simulink model "vhs_fpga_rx_to_sdram_time_share_agc_cfo"  (Simulink 7.1)
settings: Solver=FixedStepDiscrete  SolverMode=SingleTasking  StartTime=0.0  StopTime=inf  RelTol=1e-3
values from neighbouring files (symbols this model uses):
  N_FB_RX_frame = 390    [OFDM_Parameter.mat]
  Nfft = 64    [OFDM_Parameter.mat]
  Nguard = 16    [OFDM_Parameter.mat]
  Nofdm = 130    [OFDM_Parameter.mat]
  Nskip = 8    [OFDM_Parameter.mat]
undefined symbols (not defined in the file or in its folder): Fs, Sincos_Bits, Sincos_Len, Theta_Bits
libraries: xbsIndex_r4 x366, vhsadac_common_ob_fpgalib_v1_2_0 x18, misc_tools_fpgalib_v1_0_0 x6, rffe_fpgalib_v1_1_0 x1, rtdex_fpgalib_v1_1_0 x1
(part 1 of 5)
settings Model: Creator=Administrator  LastModifiedBy=lyrtech

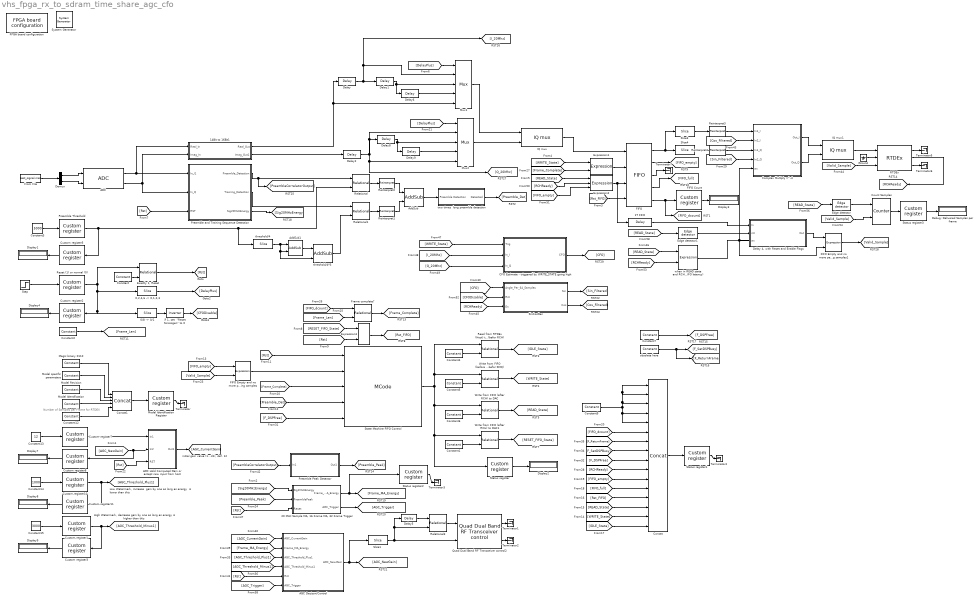
== system vhs_fpga_rx_to_sdram_time_share_agc_cfo ==
  note: Number of Samples per Frame for RTDEX
  " System Generator" : xbsIndex_r4/ System Generator  Tag=genX  SystemSampleTime=-1  xilinxfamily=virtex4  part=xc4vsx55  speed=-10  package=ff1148  synthesis_tool=XST  clock_wrapper=Clock Enables  directory=./netlist  testbench=off  simulink_period=1  sysclk_period=9  dcm_input_clock_period=100  incr_netlist=off  trim_vbits=Everywhere in SubSystem  dbl_ovrd=According to Block Masks  core_generation=According to Block Masks  run_coregen=off  deprecated_control=off  eval_field=0  block_type=sysgen
      settings: block_version=10.1.3
  "0,2,4,6 -> 0,1,2,3" : xbsIndex_r4/Slice  nbits=2  boolean_output=off  mode=Lower Bit Location + Width  bit1=0  base1=MSB of Input  bit0=1  base0=LSB of Input  dbl_ovrd=off  block_type=slice
      settings: infoedit="Extracts a given range of bits from each input sample and presents it at the output.  The output type is ordinarily unsigned with binary point at zero, but can be Boolean when the slice is one bit wide.<P><P>Hardware notes: In hardware this block costs nothing."  block_version=10.1.3
  "0/8 -> 0/1" : xbsIndex_r4/Slice  nbits=1  boolean_output=on  mode=Lower Bit Location + Width  bit1=0  base1=MSB of Input  bit0=3  base0=LSB of Input  dbl_ovrd=off  block_type=slice
      settings: infoedit="Extracts a given range of bits from each input sample and presents it at the output.  The output type is ordinarily unsigned with binary point at zero, but can be Boolean when the slice is one bit wide.<P><P>Hardware notes: In hardware this block costs nothing."  block_version=10.1.3
  14Bit to 16Bit1 : Subsystem
  1T FIFO : xbsIndex_r4/Delay  en=off  latency=1  dbl_ovrd=off  reg_retiming=off  block_type=delay
  "20 MHz Sample MA, 16 Frame MA, 32 Frame Trigger" : Subsystem
  ADC : vhsadac_common_ob_fpgalib_v1_2_0/ADC  Tag=LYR_FPGA_IO_ADC  Description=Lyrtech block  SystemSampleTime=-1  nbofcha=2  binpt=0  sample_period=5  ovr_flag=off  trig_sig=off
  AGC Decison/Control : Subsystem
  AGC Hold Computed Gain or accept new input from host : Subsystem
  AddSub : xbsIndex_r4/AddSub  mode=Addition  use_carryin=off  use_carryout=off  en=off  latency=0  precision=Full  arith_type=Unsigned  n_bits=16  bin_pt=14  quantization=Truncate  overflow=Wrap  dbl_ovrd=off  use_behavioral_HDL=off  pipelined=off  use_rpm=on  hw_selection=Fabric  block_type=addsub
      settings: block_version=10.1.3
  AddSub1 : xbsIndex_r4/AddSub  mode=Addition  use_carryin=off  use_carryout=off  en=off  latency=1  precision=Full  arith_type=Unsigned  n_bits=16  bin_pt=14  quantization=Truncate  overflow=Wrap  dbl_ovrd=off  use_behavioral_HDL=off  pipelined=off  use_rpm=on  hw_selection=Fabric  block_type=addsub
      settings: block_version=10.1.3
  CFO Estimate - triggered by WRITE_STATE going high : Subsystem
  Complex Multiply z^-4 : Subsystem
  Concat : xbsIndex_r4/Concat  num_inputs=16  dbl_ovrd=off  block_type=concat
      settings: block_version=10.1.3
  Concat1 : xbsIndex_r4/Concat  num_inputs=5  dbl_ovrd=off  block_type=concat
      settings: block_version=10.1.3
  Constant : xbsIndex_r4/Constant  arith_type=Unsigned  const=1  n_bits=32  bin_pt=0  explicit_period=on  period=5  equ=P=C  opselect=C  inp2=PCIN>>17  opr=+  inp1=P  carry=CIN  dbl_ovrd=off  block_type=constant
  Constant1 : xbsIndex_r4/Constant  arith_type=Unsigned  const=4  n_bits=3  bin_pt=0  explicit_period=on  period=5  equ=P=C  opselect=C  inp2=PCIN>>17  opr=+  inp1=P  carry=CIN  dbl_ovrd=off  block_type=constant
  Constant12 : xbsIndex_r4/Constant  arith_type=Unsigned  const=N_FB_RX_frame  n_bits=15  bin_pt=0  explicit_period=on  period=1  equ=P=C  opselect=C  inp2=PCIN>>17  opr=+  inp1=P  carry=CIN  dbl_ovrd=off  block_type=constant
  Constant13 : Constant  Value=12  OutDataType=sfix(16)  OutScaling=2^0  SampleTime=5
  Constant14 : Constant  Value=1000  OutDataType=sfix(16)  OutScaling=2^0  SampleTime=5
  Constant15 : Constant  Value=3000  OutDataType=sfix(16)  OutScaling=2^0  SampleTime=5
  Constant2 : xbsIndex_r4/Constant  arith_type=Unsigned  const=(Nfft + Nguard) * ( 1 + Nofdm )  n_bits=32  bin_pt=0  explicit_period=on  period=5  equ=P=C  opselect=C  inp2=PCIN>>17  opr=+  inp1=P  carry=CIN  dbl_ovrd=off  block_type=constant
  Constant3 : Constant  Value=5000  OutDataType=sfix(16)  OutScaling=2^0  SampleTime=5
  Constant4 : xbsIndex_r4/Constant  arith_type=Unsigned  const=1  n_bits=3  bin_pt=0  explicit_period=on  period=5  equ=P=C  opselect=C  inp2=PCIN>>17  opr=+  inp1=P  carry=CIN  dbl_ovrd=off  block_type=constant
  Constant5 : xbsIndex_r4/Constant  arith_type=Unsigned  const=2  n_bits=3  bin_pt=0  explicit_period=on  period=5  equ=P=C  opselect=C  inp2=PCIN>>17  opr=+  inp1=P  carry=CIN  dbl_ovrd=off  block_type=constant
  Constant6 : xbsIndex_r4/Constant  arith_type=Unsigned  const=3  n_bits=3  bin_pt=0  explicit_period=on  period=5  equ=P=C  opselect=C  inp2=PCIN>>17  opr=+  inp1=P  carry=CIN  dbl_ovrd=off  block_type=constant
  Constant7 : xbsIndex_r4/Constant  arith_type=Boolean  const=1  n_bits=3  bin_pt=0  explicit_period=on  period=5  equ=P=C  opselect=C  inp2=PCIN>>17  opr=+  inp1=P  carry=CIN  dbl_ovrd=off  block_type=constant
  Constant9 : xbsIndex_r4/Constant  arith_type=Unsigned  const=0  n_bits=1  bin_pt=0  explicit_period=on  period=5  equ=P=C  opselect=C  inp2=PCIN>>17  opr=+  inp1=P  carry=CIN  dbl_ovrd=off  block_type=constant
  Count Samples : xbsIndex_r4/Counter  cnt_type=Free Running  cnt_to=Inf  operation=Up  start_count=0  cnt_by_val=1  arith_type=Unsigned  n_bits=16  bin_pt=0  load_pin=off  rst=on  en=on  explicit_period=on  period=5  dbl_ovrd=off  use_behavioral_HDL=off  use_rpm=off  implementation=Fabric  block_type=counter
      settings: block_version=VER_STRING_GOES_HERE
  Custom register1 : vhsadac_common_ob_fpgalib_v1_2_0/Custom register  Tag=LYR_FPGA_IO_CUSTOM_REGISTER  Description=Lyrtech block  SystemSampleTime=-1  regID=10  direction=Read  output_arithmetic_type=Unsigned  output_width=32  binpt=0  sample_period=5
  Custom register10 : vhsadac_common_ob_fpgalib_v1_2_0/Custom register  Tag=LYR_FPGA_IO_CUSTOM_REGISTER  Description=Lyrtech block  SystemSampleTime=-1  regID=9  direction=Read  output_arithmetic_type=Unsigned  output_width=32  binpt=0  sample_period=5
  Custom register11 : vhsadac_common_ob_fpgalib_v1_2_0/Custom register  Tag=LYR_FPGA_IO_CUSTOM_REGISTER  Description=Lyrtech block  Orientation=left  SystemSampleTime=-1  regID=9  direction=Write  output_arithmetic_type=Unsigned  output_width=32  binpt=0  sample_period=5
  Custom register2 : vhsadac_common_ob_fpgalib_v1_2_0/Custom register  Tag=LYR_FPGA_IO_CUSTOM_REGISTER  Description=Lyrtech block  Orientation=left  SystemSampleTime=-1  regID=2  direction=Write  output_arithmetic_type=Unsigned  output_width=32  binpt=0  sample_period=5
  Custom register3 : vhsadac_common_ob_fpgalib_v1_2_0/Custom register  Tag=LYR_FPGA_IO_CUSTOM_REGISTER  Description=Lyrtech block  Orientation=left  SystemSampleTime=-1  regID=10  direction=Write  output_arithmetic_type=Unsigned  output_width=32  binpt=0  sample_period=5
  Custom register5 : vhsadac_common_ob_fpgalib_v1_2_0/Custom register  Tag=LYR_FPGA_IO_CUSTOM_REGISTER  Description=Lyrtech block  Orientation=left  SystemSampleTime=-1  regID=1  direction=Write  output_arithmetic_type=Unsigned  output_width=32  binpt=0  sample_period=5
  Custom register7 : vhsadac_common_ob_fpgalib_v1_2_0/Custom register  Tag=LYR_FPGA_IO_CUSTOM_REGISTER  Description=Lyrtech block  SystemSampleTime=-1  regID=8  direction=Read  output_arithmetic_type=Unsigned  output_width=32  binpt=0  sample_period=5
  Custom register8 : vhsadac_common_ob_fpgalib_v1_2_0/Custom register  Tag=LYR_FPGA_IO_CUSTOM_REGISTER  Description=Lyrtech block  Orientation=left  SystemSampleTime=-1  regID=8  direction=Write  output_arithmetic_type=Unsigned  output_width=32  binpt=0  sample_period=5
  Debug: Delivered Samples per frame : Display
  Delay : xbsIndex_r4/Delay  en=off  latency=106  dbl_ovrd=off  reg_retiming=off  block_type=delay
  "Delay 4, with Reset and Enable Flags" : Subsystem
  Delay{1,5..6,8..9} (5 alike) : xbsIndex_r4/Delay  en=off  latency=1  dbl_ovrd=off  reg_retiming=off  block_type=delay
  Delay2 : xbsIndex_r4/Delay  en=off  latency=106  dbl_ovrd=off  reg_retiming=off  block_type=delay
  Demux : Demux  Outputs=2
  Display{1..4,7..9} (7 alike) : Display
  Edge detector : misc_tools_fpgalib_v1_0_0/Edge detector  Tag=LYR_FPGA_MISC_EDGE_DETECTOR  Description=Lyrtech block  SystemSampleTime=-1  edge_detect=Rising  and_latency=0
  Edge detector1 : misc_tools_fpgalib_v1_0_0/Edge detector  Tag=LYR_FPGA_MISC_EDGE_DETECTOR  Description=Lyrtech block  SystemSampleTime=-1  edge_detect=Rising  and_latency=0
  "Exactly 1, Reset" : xbsIndex_r4/Relational  mode=a=b  en=off  latency=1  dbl_ovrd=off  block_type=relational
      settings: block_version=10.1.3
  Expression1 : xbsIndex_r4/Expression  expression=a & ~b  align_bp=on  en=off  latency=0  precision=Full  arith_type=Unsigned  n_bits=16  bin_pt=0  dbl_ovrd=off  block_type=expr
      settings: block_version=10.1.3
  Expression2 : xbsIndex_r4/Expression  expression=a & b & ~c  align_bp=on  en=off  latency=0  precision=Full  arith_type=Unsigned  n_bits=16  bin_pt=0  dbl_ovrd=off  block_type=expr
      settings: block_version=10.1.3
  Expression3 : xbsIndex_r4/Expression  expression=a | b  align_bp=on  en=off  latency=0  precision=Full  arith_type=Unsigned  n_bits=16  bin_pt=0  dbl_ovrd=off  block_type=expr
      settings: block_version=10.1.3
  FIFO : xbsIndex_r4/FIFO  depth=16K  percent_nbits=1  rst=on  en=off  use_dcount=on  use_almost_empty=off  almost_empty_thresh=2  use_almost_full=off  almost_full_thresh=14  dbl_ovrd=off  mem_type=Block RAM  block_type=fifo
      settings: block_version=10.1.3
  FIFO Count : vhsadac_common_ob_fpgalib_v1_2_0/Custom register  Tag=LYR_FPGA_IO_CUSTOM_REGISTER  Description=Lyrtech block  SystemSampleTime=-1  regID=3  direction=Write  output_arithmetic_type=Unsigned  output_width=32  binpt=0  sample_period=5
  FIFO Empty and no more pending samples : xbsIndex_r4/Expression  expression=a & ~b  align_bp=on  en=off  latency=0  precision=Full  arith_type=Unsigned  n_bits=16  bin_pt=0  dbl_ovrd=off  block_type=expr
      settings: block_version=10.1.3
  FIFO Empty and no more pending samples1 : xbsIndex_r4/Expression  expression=a & b  align_bp=on  en=off  latency=0  precision=Full  arith_type=Unsigned  n_bits=16  bin_pt=0  dbl_ovrd=off  block_type=expr
      settings: block_version=10.1.3
  FPGA board configuration : vhsadac_common_ob_fpgalib_v1_2_0/FPGA board configuration  Tag=SysgenCompile  Description=Lyrtech block  SystemSampleTime=-1  clk_sel=Hardware implementation  clk_src=ADC/DAC clock  hardware=VHS-ADC Virtex-4  copy_bit_cd=on
  Frame complete? : xbsIndex_r4/Relational  mode=a>=b  en=off  latency=0  dbl_ovrd=off  block_type=relational
      settings: block_version=10.1.3
  From File : FromFile  FileName=test_signal.mat  SampleTime=5
  Ground : Ground
  IQ mux : misc_tools_fpgalib_v1_0_0/IQ mux  Tag=LYR_FPGA_MISC_IQ_MUX  Description=Lyrtech block  SystemSampleTime=-1
  IQ mux1 : misc_tools_fpgalib_v1_0_0/IQ mux  Tag=LYR_FPGA_MISC_IQ_MUX  Description=Lyrtech block  SystemSampleTime=-1
  Magic binary 0110 : xbsIndex_r4/Constant  arith_type=Unsigned  const=6  n_bits=4  bin_pt=0  explicit_period=on  period=1  equ=P=C  opselect=C  inp2=PCIN>>17  opr=+  inp1=P  carry=CIN  dbl_ovrd=off  block_type=constant
  Model Identification : xbsIndex_r4/Constant  arith_type=Unsigned  const=1  n_bits=4  bin_pt=0  explicit_period=on  period=1  equ=P=C  opselect=C  inp2=PCIN>>17  opr=+  inp1=P  carry=CIN  dbl_ovrd=off  block_type=constant
  Model Identification Register : vhsadac_common_ob_fpgalib_v1_2_0/Custom register  Tag=LYR_FPGA_IO_CUSTOM_REGISTER  Description=Lyrtech block  SystemSampleTime=-1  regID=7  direction=Write  output_arithmetic_type=Unsigned  output_width=32  binpt=0  sample_period=1
  Model Revision : xbsIndex_r4/Constant  arith_type=Unsigned  const=2  n_bits=3  bin_pt=0  explicit_period=on  period=1  equ=P=C  opselect=C  inp2=PCIN>>17  opr=+  inp1=P  carry=CIN  dbl_ovrd=off  block_type=constant
  Model specific parameters : xbsIndex_r4/Constant  arith_type=Unsigned  const=0  n_bits=6  bin_pt=0  explicit_period=on  period=1  equ=P=C  opselect=C  inp2=PCIN>>17  opr=+  inp1=P  carry=CIN  dbl_ovrd=off  block_type=constant
  Mux1 : xbsIndex_r4/Mux  inputs=4  en=off  latency=0  precision=Full  arith_type=Unsigned  n_bits=16  bin_pt=14  quantization=Truncate  overflow=Wrap  dbl_ovrd=off  block_type=mux
  Mux2 : xbsIndex_r4/Mux  inputs=4  en=off  latency=0  precision=Full  arith_type=Unsigned  n_bits=16  bin_pt=14  quantization=Truncate  overflow=Wrap  dbl_ovrd=off  block_type=mux
  Preamble Peak Detector : Subsystem
  Preamble Threshold : vhsadac_common_ob_fpgalib_v1_2_0/Custom register  Tag=LYR_FPGA_IO_CUSTOM_REGISTER  Description=Lyrtech block  SystemSampleTime=-1  regID=1  direction=Read  output_arithmetic_type=Unsigned  output_width=32  binpt=0  sample_period=5
  Preamble and Training Sequence Detection : Subsystem
  Quad Dual Band RF Transceiver control2 : rffe_fpgalib_v1_1_0/Quad Dual Band RF Transceiver control  Tag=LYR_FPGA_CONTROL_QUAD_DUAL_BAND_RF_TRANSCEIVER_CONTROL  Description=Lyrtech block  SystemSampleTime=-1  external_gain=on  tx1=off  tx2=off  tx3=off  tx4=off  mode=off  add=off  int_divider=off  frac_divider=off  int_divider_en=off  frac_divider_en=off  lock_detect=off  sample_period=5
  RTDEx : rtdex_fpgalib_v1_1_0/RTDEx  Tag=LYR_FPGA_IO_RTDEX  Description=Lyrtech block  SystemSampleTime=-1  direction=TX  output_arithmetic_type=Unsigned  output_width=32  binpt=0  provide_control=off  sample_period=5
  Read from RTDEx (Host) to FIFO (befor RCH) : xbsIndex_r4/Relational  mode=a=b  en=off  latency=0  dbl_ovrd=off  block_type=relational
      settings: block_version=10.1.3
  Reinterpret1 : xbsIndex_r4/Reinterpret  force_arith_type=on  arith_type=Unsigned  force_bin_pt=on  bin_pt=0  block_type=reinterpret
      settings: infoedit="Changes signal type without altering the binary representation.   You can changed the signal between signed and unsigned, and relocate the binary point.<P><P>Hardware notes: In hardware this block costs nothing.<P><P>Example:  Suppose the input is 6 bits wide, signed, with 2 fractional bits, and the output is forced to unsigned with 0 fractional bits.  Then an input of -2.0 (1110.00 in binary 2's complement) becomes an output of 56 (111000 in binary)."  block_version=10.1.3
  Reinterpret2 : xbsIndex_r4/Reinterpret  force_arith_type=on  arith_type=Unsigned  force_bin_pt=on  bin_pt=0  block_type=reinterpret
      settings: infoedit="Changes signal type without altering the binary representation.   You can changed the signal between signed and unsigned, and relocate the binary point.<P><P>Hardware notes: In hardware this block costs nothing.<P><P>Example:  Suppose the input is 6 bits wide, signed, with 2 fractional bits, and the output is forced to unsigned with 0 fractional bits.  Then an input of -2.0 (1110.00 in binary 2's complement) becomes an output of 56 (111000 in binary)."  block_version=10.1.3
  Reinterpret3 : xbsIndex_r4/Reinterpret  force_arith_type=on  arith_type="Signed  (2's comp)"  force_bin_pt=on  bin_pt=0  block_type=reinterpret
      settings: infoedit="Changes signal type without altering the binary representation.   You can changed the signal between signed and unsigned, and relocate the binary point.<P><P>Hardware notes: In hardware this block costs nothing.<P><P>Example:  Suppose the input is 6 bits wide, signed, with 2 fractional bits, and the output is forced to unsigned with 0 fractional bits.  Then an input of -2.0 (1110.00 in binary 2's complement) becomes an output of 56 (111000 in binary)."  block_version=10.1.3
  Reinterpret4 : xbsIndex_r4/Reinterpret  force_arith_type=on  arith_type="Signed  (2's comp)"  force_bin_pt=on  bin_pt=0  block_type=reinterpret
      settings: infoedit="Changes signal type without altering the binary representation.   You can changed the signal between signed and unsigned, and relocate the binary point.<P><P>Hardware notes: In hardware this block costs nothing.<P><P>Example:  Suppose the input is 6 bits wide, signed, with 2 fractional bits, and the output is forced to unsigned with 0 fractional bits.  Then an input of -2.0 (1110.00 in binary 2's complement) becomes an output of 56 (111000 in binary)."  block_version=10.1.3
  Relational : xbsIndex_r4/Relational  mode=a>=b  en=off  latency=1  dbl_ovrd=off  block_type=relational
      settings: block_version=10.1.3
  Relational1 : xbsIndex_r4/Relational  mode=a>=b  en=off  latency=1  dbl_ovrd=off  block_type=relational
      settings: block_version=10.1.3
  Relational3 : xbsIndex_r4/Relational  mode=a!=b  en=off  latency=1  dbl_ovrd=off  block_type=relational
      settings: block_version=10.1.3
  Reset (1) or normal (0) : vhsadac_common_ob_fpgalib_v1_2_0/Custom register  Tag=LYR_FPGA_IO_CUSTOM_REGISTER  Description=Lyrtech block  SystemSampleTime=-1  regID=2  direction=Read  output_arithmetic_type=Unsigned  output_width=32  binpt=0  sample_period=5
  SinCosGen : Subsystem
  Slice1 : xbsIndex_r4/Slice  nbits=7  boolean_output=off  mode=Lower Bit Location + Width  bit1=0  base1=MSB of Input  bit0=0  base0=LSB of Input  dbl_ovrd=off  block_type=slice
      settings: infoedit="Extracts a given range of bits from each input sample and presents it at the output.  The output type is ordinarily unsigned with binary point at zero, but can be Boolean when the slice is one bit wide.<P><P>Hardware notes: In hardware this block costs nothing."  block_version=10.1.3
  Slice3 : xbsIndex_r4/Slice  nbits=16  boolean_output=off  mode=Upper Bit Location + Width  bit1=0  base1=MSB of Input  bit0=0  base0=LSB of Input  dbl_ovrd=off  block_type=slice
      settings: infoedit="Extracts a given range of bits from each input sample and presents it at the output.  The output type is ordinarily unsigned with binary point at zero, but can be Boolean when the slice is one bit wide.<P><P>Hardware notes: In hardware this block costs nothing."  block_version=10.1.3
  Slice4 : xbsIndex_r4/Slice  nbits=16  boolean_output=off  mode=Lower Bit Location + Width  bit1=0  base1=MSB of Input  bit0=0  base0=LSB of Input  dbl_ovrd=off  block_type=slice
      settings: infoedit="Extracts a given range of bits from each input sample and presents it at the output.  The output type is ordinarily unsigned with binary point at zero, but can be Boolean when the slice is one bit wide.<P><P>Hardware notes: In hardware this block costs nothing."  block_version=10.1.3
  State Machine FIFO Control : xbsIndex_r4/MCode  mfname=vhs_state_machine_fifo  explicit_period=on  period=5  inputsTable={'boundInpExpr'=>['','','','',''],'inputs'=>['RST','FIFO_Empty','FIFO_Filled','Preamble_Det','DSPFree']}  outputsTable={'outputs'=>['sel'],'suppressOut'=>['off']}  dbl_ovrd=off  enable_stdout=off  enable_debug=off  suppress_output=1  defparams={}  hide_port_list={}  block_type=mcode
      settings: block_version=10.1.3
  Status register : vhsadac_common_ob_fpgalib_v1_2_0/Custom register  Tag=LYR_FPGA_IO_CUSTOM_REGISTER  Description=Lyrtech block  SystemSampleTime=-1  regID=0  direction=Write  output_arithmetic_type=Unsigned  output_width=32  binpt=0  sample_period=5
  Status register1 : vhsadac_common_ob_fpgalib_v1_2_0/Custom register  Tag=LYR_FPGA_IO_CUSTOM_REGISTER  Description=Lyrtech block  SystemSampleTime=-1  regID=5  direction=Write  output_arithmetic_type=Unsigned  output_width=32  binpt=0  sample_period=5
  Status register2 : vhsadac_common_ob_fpgalib_v1_2_0/Custom register  Tag=LYR_FPGA_IO_CUSTOM_REGISTER  Description=Lyrtech block  SystemSampleTime=-1  regID=11  direction=Write  output_arithmetic_type=Unsigned  output_width=32  binpt=0  sample_period=5
  Status register3 : vhsadac_common_ob_fpgalib_v1_2_0/Custom register  Tag=LYR_FPGA_IO_CUSTOM_REGISTER  Description=Lyrtech block  SystemSampleTime=-1  regID=6  direction=Write  output_arithmetic_type=Unsigned  output_width=32  binpt=0  sample_period=5
  Step : Step  Time=5  Before=1  After=0  SampleTime=5
  Terminator{,1..7} (8 alike) : Terminator
  Write from FIFO (after RCH) to DAC : xbsIndex_r4/Relational  mode=a=b  en=off  latency=0  dbl_ovrd=off  block_type=relational
      settings: block_version=10.1.3
  Write from FIFO (after RCH) to DAC1 : xbsIndex_r4/Relational  mode=a=b  en=off  latency=0  dbl_ovrd=off  block_type=relational
      settings: block_version=10.1.3
  Write from FIFO (before RCH) to RCH (befor SMQ) : xbsIndex_r4/Relational  mode=a=b  en=off  latency=0  dbl_ovrd=off  block_type=relational
      settings: block_version=10.1.3
  "if 1, set  \"Reset Sincosgen\" to 0" : xbsIndex_r4/Inverter  en=off  latency=0  dbl_ovrd=off  block_type=inv
  obsolete here : xbsIndex_r4/Constant  arith_type=Boolean  const=0  n_bits=3  bin_pt=0  explicit_period=on  period=5  equ=P=C  opselect=C  inp2=PCIN>>17  opr=+  inp1=P  carry=CIN  dbl_ovrd=off  block_type=constant
  threshold/4 : xbsIndex_r4/Slice  nbits=30  boolean_output=off  mode=Upper Bit Location + Width  bit1=0  base1=MSB of Input  bit0=0  base0=LSB of Input  dbl_ovrd=off  block_type=slice
      settings: infoedit="Extracts a given range of bits from each input sample and presents it at the output.  The output type is ordinarily unsigned with binary point at zero, but can be Boolean when the slice is one bit wide.<P><P>Hardware notes: In hardware this block costs nothing."  block_version=10.1.3
  threshold/4*3 : xbsIndex_r4/AddSub  mode=Addition  use_carryin=off  use_carryout=off  en=off  latency=1  precision=Full  arith_type=Unsigned  n_bits=16  bin_pt=14  quantization=Truncate  overflow=Wrap  dbl_ovrd=off  use_behavioral_HDL=off  pipelined=off  use_rpm=on  hw_selection=Fabric  block_type=addsub
      settings: block_version=10.1.3
  two times  long preamble detection : Subsystem
  "when in READ state and RCH/RTDEx willing to receive, let MPY run with 1T latency (due to FIFO latency)" : xbsIndex_r4/Expression  expression=a & b  align_bp=on  en=off  latency=1  precision=Full  arith_type=Unsigned  n_bits=16  bin_pt=0  dbl_ovrd=off  block_type=expr
      settings: block_version=10.1.3
  wires:
  From File/1 -> Demux/1
  Demux/1 -> ADC/1
  Demux/2 -> ADC/2
  Preamble Threshold/1 -> Custom register5/1, Relational/2, threshold/4/1
  Constant3/1 -> Preamble Threshold/1
  Custom register5/1 -> Display1/1
  ADC/1 -> Preamble and Training Sequence Detection/1(In_I1), 14Bit to 16Bit1/1(Real_In)
  ADC/2 -> 14Bit to 16Bit1/2(Imag_In), Preamble and Training Sequence Detection/2(In_Q)
  Preamble and Training Sequence Detection/1(Preamble_Detection) -> [PreambleCorrelatorOutput], Relational/1
  Preamble and Training Sequence Detection/2(Training_Detection) -> Relational1/1
  Relational/1 -> Reinterpret2/1
  Relational1/1 -> Reinterpret1/1
  AddSub/1 -> two times  long preamble detection/1(Preamble Detection)
  Reinterpret2/1 -> AddSub/1
  Reinterpret1/1 -> AddSub/2
  two times  long preamble detection/1(Detected) -> [Preamble_Det]
  Delay/1 -> Delay1/1, Mux1/2, [I_20Mhz]
  Reset (1) or normal (0)/1 -> "Exactly 1, Reset"/1, "0,2,4,6 -> 0,1,2,3"/1, Custom register2/1, "0/8 -> 0/1"/1
  "Exactly 1, Reset"/1 -> [Rst]
  Constant/1 -> "Exactly 1, Reset"/2
  Step/1 -> Reset (1) or normal (0)/1
  IQ mux/1 -> FIFO/1
  FIFO/5 -> FIFO Count/1, [FIFO_dcount]
  FIFO Count/1 -> Display3/1
  Constant4/1 -> Read from RTDEx (Host) to FIFO (befor RCH)/2
  Constant5/1 -> Write from FIFO (before RCH) to RCH (befor SMQ)/2
  Read from RTDEx (Host) to FIFO (befor RCH)/1 -> [IDLE_State]
  Write from FIFO (before RCH) to RCH (befor SMQ)/1 -> [WRITE_State]
  Write from FIFO (after RCH) to DAC/1 -> [READ_State]
  Constant6/1 -> Write from FIFO (after RCH) to DAC/2
  Status register/1 -> Display2/1
  Custom register2/1 -> Display4/1
  [Rst_FIFO] -> FIFO/4
  [WRITE_State] -> Expression1/1
  Expression1/1 -> FIFO/2
  FIFO/4 -> [FIFO_full]
  Expression2/1 -> FIFO/3, 1T FIFO/1
  [READ_State] -> Expression2/1
  FIFO/2 -> [FIFO_empty]
  [Rst] -> Preamble and Training Sequence Detection/3(RST)
  14Bit to 16Bit1/1(Real_Out) -> Delay/1, Mux1/5
  14Bit to 16Bit1/2(Imag_Out1) -> Delay2/1
  Write from FIFO (after RCH) to DAC1/1 -> [RESET_FIFO_State]
  Constant1/1 -> Write from FIFO (after RCH) to DAC1/2
  Expression3/1 -> [Rst_FIFO]
  [RESET_FIFO_State] -> Expression3/1
  [Rst] -> Expression3/2
  [Rst] -> State Machine FIFO Control/1
  [Frame_Complete] -> State Machine FIFO Control/3
  [Preamble_Det] -> State Machine FIFO Control/4
  State Machine FIFO Control/1 -> Write from FIFO (after RCH) to DAC1/1, Status register/1, Write from FIFO (after RCH) to DAC/1, Write from FIFO (before RCH) to RCH (befor SMQ)/1, Read from RTDEx (Host) to FIFO (befor RCH)/1
  Concat/1 -> Status register1/1
  Constant2/1 -> [Frame_Len]
  Frame complete?/1 -> [Frame_Complete]
  [Frame_Complete] -> Expression1/2
  [Frame_Len] -> Frame complete?/2
  [FIFO_dcount] -> Frame complete?/1
  [IDLE_State] -> Concat/16
  [WRITE_State] -> Concat/15
  [READ_State] -> Concat/14
  [Rst_FIFO] -> Concat/13
  [FIFO_full] -> Concat/12
  [FIFO_empty] -> Concat/11
  [RCHReady] -> Concat/10
  Constant9/1 -> Concat/1, Concat/2, Concat/3, Concat/4, Concat/5
  [F_DSPFree] -> State Machine FIFO Control/5
  [F_DSPFree] -> Concat/9
  [F_SetDSPBusy] -> Concat/8
  [F_ReturnFrame] -> Concat/7
  [FIFO_dcount] -> Concat/6
  Concat1/1 -> Model Identification Register/1
  Constant12/1 -> Concat1/5
  Model Identification/1 -> Concat1/4
  Model Revision/1 -> Concat1/3
  Model specific parameters/1 -> Concat1/2
  Magic binary 0110/1 -> Concat1/1
  Constant13/1 -> Custom register7/1
  Custom register8/1 -> Display7/1
  Custom register10/1 -> Custom register11/1, [AGC_Threshold_Plus1]
  Constant14/1 -> Custom register10/1
  Custom register11/1 -> Display8/1
  Custom register1/1 -> Custom register3/1, [AGC_Threshold_Minus1]
  Constant15/1 -> Custom register1/1
  Custom register3/1 -> Display9/1
  [AGC_NewGain] -> Custom register8/1, AGC Hold Computed Gain or accept new input from host/2(In2)
  AGC Hold Computed Gain or accept new input from host/1(Out1) -> [AGC_CurrentGain]
  Custom register7/1 -> AGC Hold Computed Gain or accept new input from host/1(In1)
  Preamble and Training Sequence Detection/3(Sig20MHzEnergy) -> [Sig20MHzEnergy]
  Relational3/1 -> Quad Dual Band RF Transceiver control2/1
  Delay5/1 -> Relational3/1
  Slice1/1 -> Quad Dual Band RF Transceiver control2/2, Relational3/2, Delay5/1
  "20 MHz Sample MA, 16 Frame MA, 32 Frame Trigger"/1(Frame_MA_Energy) -> [Frame_MA_Energy], Status register2/1
  [Preamble_Peak] -> "20 MHz Sample MA, 16 Frame MA, 32 Frame Trigger"/2(PreamblePeak)
  [Rst] -> "20 MHz Sample MA, 16 Frame MA, 32 Frame Trigger"/3(Reset)
  [AGC_Threshold_Plus1] -> AGC Decison/Control/3(AGC_Threshold_Plus1)
  [AGC_Threshold_Minus1] -> AGC Decison/Control/4(AGC_Threshold_Minus1)
  Quad Dual Band RF Transceiver control2/1 -> Terminator1/1
  Quad Dual Band RF Transceiver control2/2 -> Terminator2/1
  [Rst] -> AGC Decison/Control/5(Rst)
  [Sig20MHzEnergy] -> "20 MHz Sample MA, 16 Frame MA, 32 Frame Trigger"/1(Sig1MHzEnergy)
  "20 MHz Sample MA, 16 Frame MA, 32 Frame Trigger"/2(AGC_Trigger) -> [AGC_Trigger]
  [AGC_CurrentGain] -> AGC Decison/Control/1(AGC_CurrentGain)
  [Frame_MA_Energy] -> AGC Decison/Control/2(Frame_MA_Energy)
  AGC Decison/Control/1(AGC_NewGain) -> [AGC_NewGain], Slice1/1
  [AGC_Trigger] -> AGC Decison/Control/6(AGC_Trigger)
  Preamble Peak Detector/1(Out1) -> [Preamble_Peak]
  [PreambleCorrelatorOutput] -> Preamble Peak Detector/1(In1)
  threshold/4/1 -> AddSub1/1, AddSub1/2, threshold/4*3/2
  AddSub1/1 -> threshold/4*3/1
  threshold/4*3/1 -> Relational1/2
  Constant7/1 -> [F_DSPFree]
  obsolete here/1 -> [F_SetDSPBusy], [F_ReturnFrame]
  "0,2,4,6 -> 0,1,2,3"/1 -> [DelayPlus]
  Delay1/1 -> Delay6/1, Mux1/3
  Delay6/1 -> Mux1/4
  Mux1/1 -> IQ mux/1
  [DelayPlus] -> Mux1/1
  Delay8/1 -> Delay9/1, Mux2/3
  Delay9/1 -> Mux2/4
  [DelayPlus] -> Mux2/1
  Delay2/1 -> Delay8/1, Mux2/2, [Q_20Mhz], Mux2/5
  Mux2/1 -> IQ mux/2
  [Rst] -> AGC Hold Computed Gain or accept new input from host/3(RST)
  [WRITE_State] -> CFO Estimate - triggered by WRITE_STATE going high/1(Trig)
  [I_20Mhz] -> CFO Estimate - triggered by WRITE_STATE going high/2(In_I)
  [Q_20Mhz] -> CFO Estimate - triggered by WRITE_STATE going high/3(In_Q)
  CFO Estimate - triggered by WRITE_STATE going high/1(CFO) -> [CFO]
  SinCosGen/1(Sin) -> [Sin_Filtered]
  SinCosGen/2(Cos) -> [Cos_Filtered]
  [CFO] -> SinCosGen/1(Angle_Per_64_Samples)
  IQ mux1/1 -> RTDEx/1
  Complex Multiply z^-4/1(Out_I) -> IQ mux1/1
  Complex Multiply z^-4/2(Out_Q) -> IQ mux1/2
  [Sin_Filtered] -> Complex Multiply z^-4/4(In2_Q)
  [Cos_Filtered] -> Complex Multiply z^-4/2(In2_I)
  FIFO/1 -> Slice4/1, Slice3/1
  Slice3/1 -> Reinterpret3/1
  Slice4/1 -> Reinterpret4/1
  [CFODisable] -> SinCosGen/2(Rst)
  [RCHReady] -> SinCosGen/3(En)
  [RCHReady] -> Expression2/2
  [FIFO_empty] -> Expression2/3
  RTDEx/2 -> [RCHReady]
  "0/8 -> 0/1"/1 -> "if 1, set  \"Reset Sincosgen\" to 0"/1
  "if 1, set  \"Reset Sincosgen\" to 0"/1 -> [CFODisable]
  Model Identification Register/1 -> Terminator/1
  Status register2/1 -> Terminator3/1
  Status register1/1 -> Terminator4/1
  RTDEx/1 -> Terminator5/1
  RTDEx/3 -> Terminator6/1
  Ground/1 -> RTDEx/2
  Reinterpret3/1 -> Complex Multiply z^-4/1(In1_I)
  Reinterpret4/1 -> Complex Multiply z^-4/3(In1_Q)
  FIFO/3 -> Terminator7/1
  FIFO Empty and no more pending samples/1 -> State Machine FIFO Control/2
  Edge detector/1 -> Count Samples/1
  [READ_State] -> Edge detector/1
  Count Samples/1 -> Status register3/1
  Status register3/1 -> Debug: Delivered Samples per frame/1
  1T FIFO/1 -> "Delay 4, with Reset and Enable Flags"/1(In)
  [READ_State] -> "when in READ state and RCH/RTDEx willing to receive, let MPY run with 1T latency (due to FIFO latency)"/1
  [RCHReady] -> "when in READ state and RCH/RTDEx willing to receive, let MPY run with 1T latency (due to FIFO latency)"/2
  "when in READ state and RCH/RTDEx willing to receive, let MPY run with 1T latency (due to FIFO latency)"/1 -> FIFO Empty and no more pending samples1/2, Complex Multiply z^-4/5(en), "Delay 4, with Reset and Enable Flags"/3(en)
  [FIFO_empty] -> FIFO Empty and no more pending samples/1
  [Valid_Sample] -> FIFO Empty and no more pending samples/2
  [Valid_Sample] -> RTDEx/3
  [Valid_Sample] -> Count Samples/2
  FIFO Empty and no more pending samples1/1 -> [Valid_Sample]
  [READ_State] -> Edge detector1/1
  Edge detector1/1 -> "Delay 4, with Reset and Enable Flags"/2(rst)
  "Delay 4, with Reset and Enable Flags"/1(Out) -> FIFO Empty and no more pending samples1/1

== system vhs_fpga_rx_to_sdram_time_share_agc_cfo/14Bit to 16Bit1 ==
  Real_In : Inport  OutDataType=sfix(16)  OutScaling=2^0
  Imag_In : Inport  Port=2  OutDataType=sfix(16)  OutScaling=2^0
  Concat : xbsIndex_r4/Concat  num_inputs=2  dbl_ovrd=off  block_type=concat
      settings: block_version=10.1.3
  Concat1 : xbsIndex_r4/Concat  num_inputs=2  dbl_ovrd=off  block_type=concat
      settings: block_version=10.1.3
  Constant : xbsIndex_r4/Constant  arith_type=Unsigned  const=0  n_bits=2  bin_pt=0  explicit_period=on  period=5  equ=P=C  opselect=C  inp2=PCIN>>17  opr=+  inp1=P  carry=CIN  dbl_ovrd=off  block_type=constant
  Constant1 : xbsIndex_r4/Constant  arith_type=Unsigned  const=0  n_bits=2  bin_pt=0  explicit_period=on  period=5  equ=P=C  opselect=C  inp2=PCIN>>17  opr=+  inp1=P  carry=CIN  dbl_ovrd=off  block_type=constant
  Reinterpret : xbsIndex_r4/Reinterpret  force_arith_type=on  arith_type="Signed  (2's comp)"  force_bin_pt=on  bin_pt=0  block_type=reinterpret
      settings: infoedit="Changes signal type without altering the binary representation.   You can changed the signal between signed and unsigned, and relocate the binary point.<P><P>Hardware notes: In hardware this block costs nothing.<P><P>Example:  Suppose the input is 6 bits wide, signed, with 2 fractional bits, and the output is forced to unsigned with 0 fractional bits.  Then an input of -2.0 (1110.00 in binary 2's complement) becomes an output of 56 (111000 in binary)."  block_version=10.1.3
  Reinterpret1 : xbsIndex_r4/Reinterpret  force_arith_type=on  arith_type="Signed  (2's comp)"  force_bin_pt=on  bin_pt=0  block_type=reinterpret
      settings: infoedit="Changes signal type without altering the binary representation.   You can changed the signal between signed and unsigned, and relocate the binary point.<P><P>Hardware notes: In hardware this block costs nothing.<P><P>Example:  Suppose the input is 6 bits wide, signed, with 2 fractional bits, and the output is forced to unsigned with 0 fractional bits.  Then an input of -2.0 (1110.00 in binary 2's complement) becomes an output of 56 (111000 in binary)."  block_version=10.1.3
  Reinterpret2 : xbsIndex_r4/Reinterpret  force_arith_type=on  arith_type=Unsigned  force_bin_pt=on  bin_pt=0  block_type=reinterpret
      settings: infoedit="Changes signal type without altering the binary representation.   You can changed the signal between signed and unsigned, and relocate the binary point.<P><P>Hardware notes: In hardware this block costs nothing.<P><P>Example:  Suppose the input is 6 bits wide, signed, with 2 fractional bits, and the output is forced to unsigned with 0 fractional bits.  Then an input of -2.0 (1110.00 in binary 2's complement) becomes an output of 56 (111000 in binary)."  block_version=10.1.3
  Reinterpret3 : xbsIndex_r4/Reinterpret  force_arith_type=on  arith_type=Unsigned  force_bin_pt=on  bin_pt=0  block_type=reinterpret
      settings: infoedit="Changes signal type without altering the binary representation.   You can changed the signal between signed and unsigned, and relocate the binary point.<P><P>Hardware notes: In hardware this block costs nothing.<P><P>Example:  Suppose the input is 6 bits wide, signed, with 2 fractional bits, and the output is forced to unsigned with 0 fractional bits.  Then an input of -2.0 (1110.00 in binary 2's complement) becomes an output of 56 (111000 in binary)."  block_version=10.1.3
  Scope6 : Scope  NumInputPorts=4
      settings: YMin=-5~-5~-5~-5  YMax=5~5~5~5  SaveName=ScopeData9  MaxDataPoints=500000
  Real_Out : Outport  OutDataType=sfix(16)  OutScaling=2^0
  Imag_Out1 : Outport  Port=2  OutDataType=sfix(16)  OutScaling=2^0
  wires:
  Reinterpret3/1 -> Concat1/1
  Constant1/1 -> Concat1/2
  Reinterpret2/1 -> Concat/1
  Constant/1 -> Concat/2
  Reinterpret1/1 -> Scope6/3, Imag_Out1/1
  Reinterpret/1 -> Scope6/1, Real_Out/1
  Concat1/1 -> Reinterpret1/1
  Concat/1 -> Reinterpret/1
  Imag_In/1 -> Reinterpret3/1, Scope6/4
  Real_In/1 -> Reinterpret2/1, Scope6/2

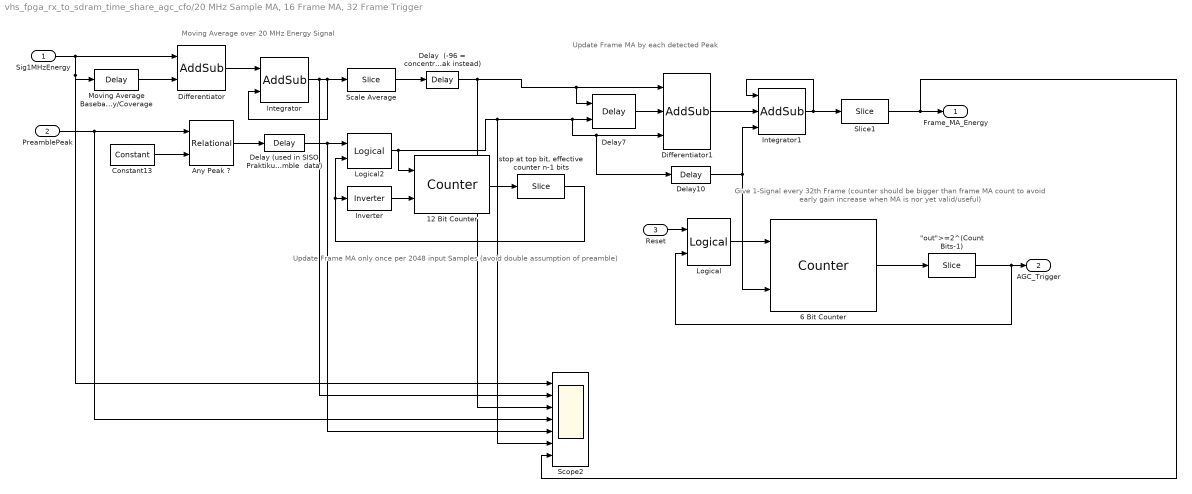
== system vhs_fpga_rx_to_sdram_time_share_agc_cfo/20 MHz Sample MA, 16 Frame MA, 32 Frame Trigger ==
  note: Moving Average over 20 MHz Energy Signal
  note: Give 1-Signal every 32th Frame
      | (counter should be bigger than frame MA count to avoid
      | early gain increase when MA is nor yet valid/useful)
  note: Update Frame MA by each detected Peak
  note: Update Frame MA only once per 2048 input Samples
      | (avoid double assumption of preamble)
  Sig1MHzEnergy : Inport
  PreamblePeak : Inport  Port=2
  Reset : Inport  Port=3
  "\"out\">=2^(Count Bits-1)" : xbsIndex_r4/Slice  nbits=1  boolean_output=on  mode=Upper Bit Location + Width  bit1=0  base1=MSB of Input  bit0=0  base0=LSB of Input  dbl_ovrd=off  block_type=slice
      settings: infoedit="Extracts a given range of bits from each input sample and presents it at the output.  The output type is ordinarily unsigned with binary point at zero, but can be Boolean when the slice is one bit wide.<P><P>Hardware notes: In hardware this block costs nothing."  block_version=10.1.3
  12 Bit Counter : xbsIndex_r4/Counter  cnt_type=Free Running  cnt_to=Inf  operation=Up  start_count=0  cnt_by_val=1  arith_type=Unsigned  n_bits=12  bin_pt=0  load_pin=off  rst=on  en=on  explicit_period=off  period=1  dbl_ovrd=off  use_behavioral_HDL=off  use_rpm=off  implementation=Fabric  block_type=counter
  6 Bit Counter : xbsIndex_r4/Counter  cnt_type=Free Running  cnt_to=Inf  operation=Up  start_count=0  cnt_by_val=1  arith_type=Unsigned  n_bits=6  bin_pt=0  load_pin=off  rst=on  en=on  explicit_period=off  period=1  dbl_ovrd=off  use_behavioral_HDL=off  use_rpm=off  implementation=Fabric  block_type=counter
  Any Peak ? : xbsIndex_r4/Relational  mode=a>=b  en=off  latency=1  dbl_ovrd=off  block_type=relational
      settings: block_version=10.1.3
  Constant13 : xbsIndex_r4/Constant  arith_type=Unsigned  const=5  n_bits=16  bin_pt=0  explicit_period=on  period=5  equ=P=C  opselect=C  inp2=PCIN>>17  opr=+  inp1=P  carry=CIN  dbl_ovrd=off  block_type=constant
  "Delay  (-96 = concentrate on STP, 0=use current position in signal->  adjust Delay for preamble peak instead)  " : xbsIndex_r4/Delay  en=off  latency=0  dbl_ovrd=off  reg_retiming=off  block_type=delay
  "Delay (used in SISO Praktikum Receiver, 0 here to concentrate  on STP if delay >0, then use some place in preamble  data)" : xbsIndex_r4/Delay  en=off  latency=16  dbl_ovrd=off  reg_retiming=off  block_type=delay
  Delay10 : xbsIndex_r4/Delay  en=off  latency=1  dbl_ovrd=off  reg_retiming=off  block_type=delay
  Delay7 : xbsIndex_r4/Delay  en=on  latency=16  dbl_ovrd=off  reg_retiming=off  block_type=delay
  Differentiator : xbsIndex_r4/AddSub  mode=Subtraction  use_carryin=off  use_carryout=off  en=off  latency=0  precision=Full  arith_type=Unsigned  n_bits=16  bin_pt=14  quantization=Truncate  overflow=Wrap  dbl_ovrd=off  use_behavioral_HDL=off  pipelined=off  use_rpm=on  hw_selection=Fabric  block_type=addsub
      settings: block_version=10.1.3
  Differentiator1 : xbsIndex_r4/AddSub  mode=Subtraction  use_carryin=off  use_carryout=off  en=on  latency=1  precision=Full  arith_type=Unsigned  n_bits=16  bin_pt=14  quantization=Truncate  overflow=Wrap  dbl_ovrd=off  use_behavioral_HDL=off  pipelined=off  use_rpm=on  hw_selection=Fabric  block_type=addsub
      settings: block_version=10.1.3
  Integrator : xbsIndex_r4/AddSub  mode=Addition  use_carryin=off  use_carryout=off  en=off  latency=1  precision=User Defined  arith_type="Signed  (2's comp)"  n_bits=22  bin_pt=0  quantization=Truncate  overflow=Saturate  dbl_ovrd=off  use_behavioral_HDL=off  pipelined=off  use_rpm=on  hw_selection=Fabric  block_type=addsub
      settings: block_version=10.1.3
  Integrator1 : xbsIndex_r4/AddSub  mode=Addition  use_carryin=off  use_carryout=off  en=on  latency=1  precision=User Defined  arith_type="Signed  (2's comp)"  n_bits=21  bin_pt=0  quantization=Truncate  overflow=Saturate  dbl_ovrd=off  use_behavioral_HDL=off  pipelined=off  use_rpm=on  hw_selection=Fabric  block_type=addsub
      settings: block_version=10.1.3
  Inverter : xbsIndex_r4/Inverter  en=off  latency=0  dbl_ovrd=off  block_type=inv
  Logical : xbsIndex_r4/Logical  logical_function=OR  inputs=2  en=off  latency=0  precision=Full  arith_type=Unsigned  n_bits=16  bin_pt=0  align_bp=on  dbl_ovrd=off  block_type=logical
  Logical2 : xbsIndex_r4/Logical  logical_function=AND  inputs=2  en=off  latency=0  precision=Full  arith_type=Unsigned  n_bits=16  bin_pt=0  align_bp=on  dbl_ovrd=off  block_type=logical
  Moving Average Baseband (20MHz) Delay/Coverage : xbsIndex_r4/Delay  en=off  latency=32  dbl_ovrd=off  reg_retiming=off  block_type=delay
  Scale Average : xbsIndex_r4/Slice  nbits=16  boolean_output=off  mode=Upper Bit Location + Width  bit1=-1  base1=MSB of Input  bit0=0  base0=LSB of Input  dbl_ovrd=off  block_type=slice
      settings: infoedit="Extracts a given range of bits from each input sample and presents it at the output.  The output type is ordinarily unsigned with binary point at zero, but can be Boolean when the slice is one bit wide.<P><P>Hardware notes: In hardware this block costs nothing."  block_version=10.1.3
  Scope2 : Scope  NumInputPorts=7
      settings: TimeRange=368.2072117826308  YMin=0~0~0~-20000~0~0~0  YMax=40000~300000~10000~40000~1~1~600  SaveName=ScopeData6  MaxDataPoints=500000
  Slice1 : xbsIndex_r4/Slice  nbits=16  boolean_output=off  mode=Upper Bit Location + Width  bit1=-1  base1=MSB of Input  bit0=0  base0=LSB of Input  dbl_ovrd=off  block_type=slice
      settings: infoedit="Extracts a given range of bits from each input sample and presents it at the output.  The output type is ordinarily unsigned with binary point at zero, but can be Boolean when the slice is one bit wide.<P><P>Hardware notes: In hardware this block costs nothing."  block_version=10.1.3
  "stop at top bit, effective counter n-1 bits" : xbsIndex_r4/Slice  nbits=1  boolean_output=on  mode=Upper Bit Location + Width  bit1=0  base1=MSB of Input  bit0=0  base0=LSB of Input  dbl_ovrd=off  block_type=slice
      settings: infoedit="Extracts a given range of bits from each input sample and presents it at the output.  The output type is ordinarily unsigned with binary point at zero, but can be Boolean when the slice is one bit wide.<P><P>Hardware notes: In hardware this block costs nothing."  block_version=10.1.3
  Frame_MA_Energy : Outport
  AGC_Trigger : Outport  Port=2
  wires:
  Moving Average Baseband (20MHz) Delay/Coverage/1 -> Differentiator/2
  Differentiator/1 -> Integrator/1
  Integrator/1 -> Integrator/2, Scale Average/1, Scope2/2
  Sig1MHzEnergy/1 -> Differentiator/1, Moving Average Baseband (20MHz) Delay/Coverage/1, Scope2/1
  Delay7/1 -> Differentiator1/2
  Scale Average/1 -> "Delay  (-96 = concentrate on STP, 0=use current position in signal->  adjust Delay for preamble peak instead)  "/1
  Delay10/1 -> Integrator1/3, 6 Bit Counter/2
  Differentiator1/1 -> Integrator1/2
  Integrator1/1 -> Integrator1/1, Slice1/1
  Any Peak ?/1 -> "Delay (used in SISO Praktikum Receiver, 0 here to concentrate  on STP if delay >0, then use some place in preamble  data)"/1
  Constant13/1 -> Any Peak ?/2
  6 Bit Counter/1 -> "\"out\">=2^(Count Bits-1)"/1
  "\"out\">=2^(Count Bits-1)"/1 -> Logical/2, AGC_Trigger/1
  Logical/1 -> 6 Bit Counter/1
  12 Bit Counter/1 -> "stop at top bit, effective counter n-1 bits"/1
  "stop at top bit, effective counter n-1 bits"/1 -> Inverter/1, Logical2/2
  Inverter/1 -> 12 Bit Counter/2
  Logical2/1 -> 12 Bit Counter/1, Delay7/2, Differentiator1/3, Delay10/1, Scope2/6
  "Delay (used in SISO Praktikum Receiver, 0 here to concentrate  on STP if delay >0, then use some place in preamble  data)"/1 -> Logical2/1, Scope2/5
  Slice1/1 -> Frame_MA_Energy/1, Scope2/7
  PreamblePeak/1 -> Any Peak ?/1, Scope2/4
  Reset/1 -> Logical/1
  "Delay  (-96 = concentrate on STP, 0=use current position in signal->  adjust Delay for preamble peak instead)  "/1 -> Delay7/1, Differentiator1/1, Scope2/3
